simulink model "MultiUAV_DroneShow"  (R2026a)
settings: Solver=ode1  StopTime=74.3333  FixedStep=Ts_sim  MaxStep=0.01  AbsTol=1e-6
PreLoadFcn:
  | setupParams
values from neighbouring files (symbols this model uses):
  arm_duration = 2    [setupParams.m]
  gnss_deny_mask = false(N_uav, 1)    [setupParams.m]
  gnss_err_gain = sqrt(1 - gnss_err_pole^2)    [setupParams.m]
  gnss_err_pole = exp(-Ts_sim / gnss_err_tau)    [setupParams.m]
  gnss_err_seed = reshape(40000 + (1:(N_uav * 3)), N_uav, 3)    [setupParams.m]
  gps_accuracy_rtk_fix = 0.02    [setupParams.m]
  gps_lock_duration = 2    [setupParams.m]
  gravity = 9.81    [setupParams.m]
  hb_period_ticks = mavlink_hb_interval / Ts_sim    (= 100)    [setupParams.m]
  init_positions = init_positions(pad_of, :)    [planShow.m]    (also in setupParams.m = plan.init_positions)
  Kd_pos = repmat([Kd_xy Kd_xy Kd_z], N_uav, 1)    [setupParams.m]
  Kff_pos = Kd_pos    [setupParams.m]
  Kp_pos = repmat([Kp_xy Kp_xy Kp_z], N_uav, 1)    [setupParams.m]
  land_end_time = plan.land_end_time    [packShowUpload.m]    (also in planShow.m = show_flight_duration + land_duration; setupParams.m)
  land_speed = cfg.land_speed    [planShow.m]
  land_start_time = show_flight_duration    [planShow.m]    (also in setupParams.m = plan.land_start_time)
  land_total_duration = land_duration + land_settle    [planShow.m]    (also in setupParams.m = plan.land_total_duration)
  mav_sys_span = 250    [setupParams.m]
  N_uav = 20    [DroneShowExample.m]    (also in packShowUpload.m = cfg.N_uav; planShow.m = cfg.N_uav; setupParams.m = 10)
  num_waypoints = length(upload_times)    [packShowUpload.m]    (also in setupParams.m = pack.num_waypoints)
  rtcm_data_bytes = 180    [setupParams.m]
  rtcm_interval = 1.0    (= 1)    [setupParams.m]
  rtcm_payload_bytes = 4 * 4 * rtk_n_sat    [setupParams.m]
  rtcm_period_ticks = rtcm_interval / Ts_sim    (= 100)    [setupParams.m]
  rtk_amb_l1_base = 1000000 + mod(97 * (1:rtk_n_sat)', 1009)    [setupParams.m]
  rtk_amb_l1_rover = rtk_amb_l1_base + rtk_amb_l1    [setupParams.m]
  rtk_amb_l2_base = 1000000 + mod(89 * (1:rtk_n_sat)', 1009)    [setupParams.m]
  rtk_amb_l2_rover = rtk_amb_l2_base + rtk_amb_l2    [setupParams.m]
  rtk_base_lla = [42.3601, -71.0589, 10]    [setupParams.m]
  rtk_deny_mask = false(N_uav, 1)    [setupParams.m]
  rtk_f1 = 1575.42e6    (= 1575420000)    [setupParams.m]
  rtk_f2 = 1227.60e6    (= 1227600000)    [setupParams.m]
  rtk_fall_slew = -gps_accuracy_standard / reconverge_time    (= -0.3)    [setupParams.m]
  rtk_fix_thresh_l1 = 0.30    (= 0.3)    [setupParams.m]
  rtk_fix_thresh_wl = 0.25    [setupParams.m]
  rtk_inject_enable = double(~skip_preflight | rtk_deny_mask(:)')    [setupParams.m]
  rtk_lambda1 = rtk_c / rtk_f1    (= 0.190293672798)    [setupParams.m]
  rtk_lambda2 = rtk_c / rtk_f2    (= 0.244210213425)    [setupParams.m]
  rtk_lambda_wl = rtk_c / (rtk_f1 - rtk_f2)    (= 0.861918400322)    [setupParams.m]
  rtk_lock_dwell = 2.0    (= 2)    [setupParams.m]
  rtk_los = [cosd(rtk_el) .* sind(rtk_az), cosd(rtk_el) .* cosd(rtk_az), sind(rtk_el)]    [setupParams.m]
  rtk_mean_clk = zeros(2, 1)    [setupParams.m]
  rtk_mean_obs = zeros(2, rtk_n_sat)    [setupParams.m]
  rtk_n_sat = numel(rtk_az)    [setupParams.m]
  rtk_rough_range = pseudoranges(rtk_base_lla, rtk_sat_pos, 'RangeAccuracy', 0)    [setupParams.m]
  rtk_sat_pos = rtk_sat_pos_all(rtk_vis, :)    [setupParams.m]
  rtk_seedm_clk = 9101 + 8 * rtk_n_sat + (0:1)'    [setupParams.m]
  rtk_seedm_l1 = rtk_seedm_p2 + 2 * rtk_n_sat    [setupParams.m]
  rtk_seedm_l2 = rtk_seedm_l1 + 2 * rtk_n_sat    [setupParams.m]
  rtk_seedm_p1 = 9101 + reshape(0:2 * rtk_n_sat - 1, 2, rtk_n_sat)    [setupParams.m]
  rtk_seedm_p2 = rtk_seedm_p1 + 2 * rtk_n_sat    [setupParams.m]
  rtk_sigma_bp = [0, rtk_timeout, rtk_float_timeout]    [setupParams.m]
  rtk_sigma_table = sqrt(max(0, rtk_sigma_tiers.^2 - gps_accuracy_rtk_fix^2))    [setupParams.m]
  rtk_sigma_unfixed = 0.75    [setupParams.m]
  rtk_slip_thresh_l1 = 0.02    [setupParams.m]
  rtk_slip_thresh_wl = 0.10    (= 0.1)    [setupParams.m]
  rtk_status_l1 = 1    [setupParams.m]
  rtk_status_unfixed = 3    [setupParams.m]
  rtk_timeout = 2.5    [setupParams.m]
  rtk_var_clk = rtk_clock_sigma^2 * ones(2, 1)    [setupParams.m]
  rtk_var_l = [rtk_sigma_phase_base^2; rtk_sigma_phase_rover^2] * ones(1, rtk_n_sat)    [setupParams.m]
  rtk_var_p = [rtk_sigma_code_base^2;  rtk_sigma_code_rover^2 ] * ones(1, rtk_n_sat)    [setupParams.m]
  skip_preflight = traj_source == 1    [DroneShowExample.m]    (also in setupParams.m = false)
  st_period_ticks = mavlink_st_interval / Ts_sim    (= 100)    [setupParams.m]
  st_phase_ticks = st_period_ticks / 2    (= 50)    [setupParams.m]
  telemetry_tx_enable = double(~skip_preflight)    [setupParams.m]
  traj_upload_flat = zeros(N_uav*num_waypoints, 7)    [packShowUpload.m]    (also in setupParams.m = pack.traj_upload_flat)
  Ts_sim = cfg.Ts_sim    [packShowUpload.m]    (also in setupParams.m = 0.01)
  uav_loss_seed = 31000 + (1:N_uav)    [setupParams.m]
  uav_mass = 0.1    [setupParams.m]
  upload_duration = (total_packets + N_uav) * Ts_sim * 1.2    [packShowUpload.m]    (also in setupParams.m = pack.upload_duration)
  upload_rate_vec = [1 ./ upload_dt; 1 / upload_dt(end)]    [packShowUpload.m]    (also in setupParams.m = pack.upload_rate_vec)
  upload_request = traj_source == 2    [DroneShowExample.m]
undefined symbols (not defined in the file or in its folder): abort_request, DiscIntNeverNeededParam, doppler, loss_seed, packet_loss_rate, Payload, SystemID, uav_loss_rate
libraries: uavmavlinklib x22, hdlsllib x16, dspsigops x8, simulink x7, matrix_library x4, commchan3 x2, etargetslib x1, uavalgslib x1, sensorinslib x1, slpidlib x1, dspmathops x1, commrandsrc3 x1
(part 2 of 4)

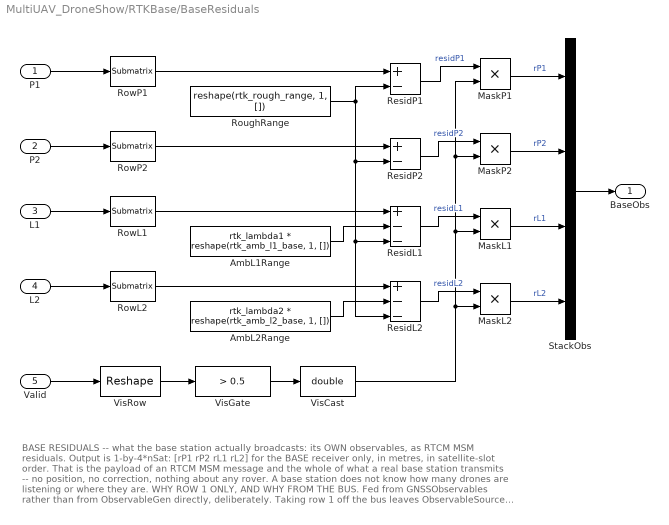
== system MultiUAV_DroneShow/RTKBase/BaseResiduals ==
  note: BASE RESIDUALS  --  what the base station actually broadcasts: its OWN observables, as RTCM MSM residuals.
      |
      | Output is 1-by-4*nSat: [rP1 rP2 rL1 rL2] for the BASE receiver only, in metres, in satellite-slot order.
      | That is the payload of an RTCM MSM message and the whole of what a real base station transmits -- no
      | position, no correction, nothing about any rover. A base station does not know how many drones are
      | listening or where they are.
      |
      | WHY ROW 1 ONLY, AND WHY FROM THE BUS. Fed from GNSSObservables rather than from ObservableGen directly,
      | deliberately. Taking row 1 off the bus leaves ObservableSource at one port, so both variant choices stay
      | identical and a RECORDING broadcasts its own base row exactly as the generator does -- the wire inherits
      | the source-agnosticism the engine itself was measured to have. Tapping ObservableGen would have added a
      | port to the Simulated choice only, and a divergence between the two choices is exactly the failure this
      | routing is arranged to make impossible.
      |
      | WHY RESIDUALS AND NOT THE OBSERVABLES. Raw values cannot survive the wire: at 2.47e7 m a single resolves
      | 2.000 m, and the payload is singles because 4*4*nSat = 128 bytes is what fits GPS_RTCM_DATA. So
      | each observable is differenced against rtk_rough_range, the clock-free noise-free base-to-satellite
      | range. A real rover can RECONSTRUCT that from the station position (RTCM 1005/1006) and the ephemeris,
      | which is what makes this a residual rather than data loss.
      |
      | WHY THE PHASE ROWS ARE ALSO CODE-ALIGNED. Subtracting the rough range alone is not enough: the base's
      | accumulated phase counter is ~1e6 cycles, so the phase residual would still sit at ~2.47e5 m, where a
      | single resolves 7.8e-3 m -- three and a half times COARSER than the 2.236e-3 m phase noise that has to
      | survive the trip. Folding the counter out here leaves ~2.3e3 m and 1.2e-4 m of resolution, nineteen times
      | finer than the noise and finer than MSM4's own 22-bit fine-phaserange field at 0.0005 m. Not a shortcut:
      | an MSM phaserange really is code-aligned, within metres of the pseudorange. The ~1e6-cycle counters are
      | RINEX semantics; this wire is RTCM semantics. Both directions were measured: residuals packed here,
      | and unpacked again the way a rover would.
      |
      | A rover differencing this recovers its OWN ambiguity rather than the between-receiver one, because the
      | base's contribution is already gone. That changes which integer a drone-side solve resolves, not whether
      | it can resolve one.
      |
      | INVISIBLE SLOTS CARRY ZERO -- that is what VisGate and the four Products are for. The payload is
      | fixed-width (nSat slots, always) because GPS_RTCM_DATA has no satellite-mask field to omit them with. An
      | unobserved slot's observable is 0 by the Valid contract, so differencing it would put -2.0e7 m on the
      | wire, indistinguishable from a catastrophically wrong residual. Masking to 0 keeps absent slots obviously
      | absent. The cost is that a slot whose residual is genuinely 0 looks absent -- a real limitation of a
      | mask-free payload, not a rounding concern: a residual is a clock plus noise, so exact 0 has measure zero.
      |
      | This was a MATLAB Function until 6-Sep-2026, and is now blocks. The replacement was accepted on two
      | measurements rather than on inspection: the block form produces bit-for-bit the same residuals the
      | function did, and at the same [1 0] rate; and the RTCM byte layout survives a round trip through these
      | very blocks. That round trip copies THIS subsystem into a throwaway model rather than restating the
      | formula anywhere it could silently drift out of step with what is built here.
  P1 : Inport
  P2 : Inport  Port=2
  L1 : Inport  Port=3
  L2 : Inport  Port=4
  Valid : Inport  Port=5
  AmbL1Range : Constant  Value=rtk_lambda1 * reshape(rtk_amb_l1_base, 1, [])  VectorParams1D=off
  AmbL2Range : Constant  Value=rtk_lambda2 * reshape(rtk_amb_l2_base, 1, [])  VectorParams1D=off
  MaskL1 : Product
  MaskL2 : Product
  MaskP1 : Product
  MaskP2 : Product
  ResidL1 : Sum  Inputs=+--
  ResidL2 : Sum  Inputs=+--
  ResidP1 : Sum  Inputs=+-
  ResidP2 : Sum  Inputs=+-
  RoughRange : Constant  Value=reshape(rtk_rough_range, 1, [])  VectorParams1D=off
  RowL1 : matrix_library/Submatrix  RowSpan=Range of rows  RowStartMode=Index  RowStartIndex=1  RowEndMode=Index  RowEndIndex=1  ColSpan=All columns  ColStartMode=First  ColStartIndex=1  ColEndMode=Last  ColEndIndex=1
  RowL2 : matrix_library/Submatrix  RowSpan=Range of rows  RowStartMode=Index  RowStartIndex=1  RowEndMode=Index  RowEndIndex=1  ColSpan=All columns  ColStartMode=First  ColStartIndex=1  ColEndMode=Last  ColEndIndex=1
  RowP1 : matrix_library/Submatrix  RowSpan=Range of rows  RowStartMode=Index  RowStartIndex=1  RowEndMode=Index  RowEndIndex=1  ColSpan=All columns  ColStartMode=First  ColStartIndex=1  ColEndMode=Last  ColEndIndex=1
  RowP2 : matrix_library/Submatrix  RowSpan=Range of rows  RowStartMode=Index  RowStartIndex=1  RowEndMode=Index  RowEndIndex=1  ColSpan=All columns  ColStartMode=First  ColStartIndex=1  ColEndMode=Last  ColEndIndex=1
  StackObs : Concatenate  NumInputs=4  Mode=Multidimensional array  ConcatenateDimension=2
  VisCast : DataTypeConversion  OutDataTypeStr=double  SaturateOnIntegerOverflow=off  RndMeth=Floor
  VisGate : simulink/Logic and Bit Operations/Compare To Constant  relop=>  const=0.5  OutDataTypeStr=boolean  ZeroCross=off
  VisRow : Reshape  OutputDimensionality=Row vector (2-D)
  BaseObs : Outport
  wires:
  P1/1 -> RowP1/1
  P2/1 -> RowP2/1
  L1/1 -> RowL1/1
  L2/1 -> RowL2/1
  Valid/1 -> VisRow/1
  VisRow/1 -> VisGate/1
  VisGate/1 -> VisCast/1
  RowP1/1 -> ResidP1/1
  RoughRange/1 -> ResidL1/3, ResidL2/3, ResidP2/2, ResidP1/2
  RowP2/1 -> ResidP2/1
  RowL1/1 -> ResidL1/1
  AmbL1Range/1 -> ResidL1/2
  RowL2/1 -> ResidL2/1
  AmbL2Range/1 -> ResidL2/2
  ResidP1/1 -> MaskP1/1  "residP1"
  VisCast/1 -> MaskP1/2, MaskP2/2, MaskL1/2, MaskL2/2
  ResidP2/1 -> MaskP2/1  "residP2"
  ResidL1/1 -> MaskL1/1  "residL1"
  ResidL2/1 -> MaskL2/1  "residL2"
  MaskP1/1 -> StackObs/1  "rP1"
  MaskP2/1 -> StackObs/2  "rP2"
  MaskL1/1 -> StackObs/3  "rL1"
  MaskL2/1 -> StackObs/4  "rL2"
  StackObs/1 -> BaseObs/1

== system MultiUAV_DroneShow/RTKBase/ObservableSource ==
  note: 1) Add Subsystem or Model blocks as valid variant choices.
      | 2) You cannot connect blocks at this level. At simulation, connectivity is automatically
      | determined, based on the active variant and port name matching.
  RoverPos : Inport
  Measured : Subsystem  Description=Recorded observables from rtk_measured_obs, e.g. a RINEX pair via rinexToObservables. The rover position input is unused here -- with real measurements the rover's truth is not known, and the observables already carry it.  VariantControl=rtk_obs_source == 2
  Simulated : Subsystem  Description=Today's simulated base station: pseudoranges() geometry, per-receiver clocks and noise, and the constellation from rtk_sat_pos.  VariantControl=rtk_obs_source == 1
  Obs : Outport

== system MultiUAV_DroneShow/RTKBase/RTKEngine ==
  Obs : Inport  Description=One epoch of raw GNSS observables, base row then rover row, metres. See createFleetBusObjects for the full contract.  OutDataTypeStr=Bus: GNSSObservableBus
  Cascade : MATLAB Function  TreatAsAtomicUnit=on
  SplitObs : BusSelector  OutputSignals=P1,P2,L1,L2,LOS,Valid
  Baseline : Outport
  Sigma : Outport  Port=2
  Status : Outport  Port=3
  Diag : Outport  Port=4
  wires:
  Cascade/1(Baseline) -> Baseline/1
  Cascade/2(Sigma) -> Sigma/1
  Cascade/3(Status) -> Status/1
  Cascade/4(Diag) -> Diag/1
  Obs/1 -> SplitObs/1
  SplitObs/1 -> Cascade/1(P1)  "<P1>"
  SplitObs/2 -> Cascade/2(P2)  "<P2>"
  SplitObs/3 -> Cascade/3(L1)  "<L1>"
  SplitObs/4 -> Cascade/4(L2)  "<L2>"
  SplitObs/5 -> Cascade/5(LOS)  "<LOS>"
  SplitObs/6 -> Cascade/6(Valid)  "<Valid>"

== system MultiUAV_DroneShow/RadioChannel/CorrectionAgeMonitor ==
  CorrAge : Inport
  GnssAvail : Inport  Port=2
  EngineSigma : Inport  Port=3
  ClampNonNegative : Saturate  UpperLimit=inf  LowerLimit=0  SampleTime=Ts_sim
  EngineGate : Product  SampleTime=Ts_sim
  EngineShortfall : Sqrt  SampleTime=Ts_sim
  EngineSigmaSq : Math  Operator=square  SampleTime=Ts_sim
  GnssAvailDbl : DataTypeConversion  OutDataTypeStr=double
  InjectEnable : Constant  Value=rtk_inject_enable
  InjectGate : Product
  InsFloorSq : Constant  Value=gps_accuracy_rtk_fix^2
  LogPosSigma : ToWorkspace  VariableName=posSigma  SaveFormat=Timeseries  SampleTime=-1
  ShortfallSq : Sum  Inputs=+-  SampleTime=Ts_sim
  SigmaGate : Product
  SigmaLUT : Lookup_n-D  NumberOfTableDimensions=1  BreakpointsForDimension1=rtk_sigma_bp  Table=rtk_sigma_table  InterpMethod=Flat  ExtrapMethod=Clip
  SigmaRateLimit : RateLimiter  RisingSlewLimit=inf  FallingSlewLimit=rtk_fall_slew  SampleTimeMode=inherited
  WorseOf : MinMax  Function=max  Inputs=2  SampleTime=Ts_sim
  PosSigma : Outport
  wires:
  InjectGate/1 -> LogPosSigma/1, PosSigma/1
  InjectEnable/1 -> InjectGate/2
  WorseOf/1 -> InjectGate/1
  CorrAge/1 -> SigmaLUT/1
  GnssAvail/1 -> GnssAvailDbl/1
  SigmaLUT/1 -> SigmaGate/1
  SigmaGate/1 -> SigmaRateLimit/1
  GnssAvailDbl/1 -> SigmaGate/2, EngineGate/2
  SigmaRateLimit/1 -> WorseOf/1
  EngineSigma/1 -> EngineSigmaSq/1
  EngineSigmaSq/1 -> ShortfallSq/1
  InsFloorSq/1 -> ShortfallSq/2
  ShortfallSq/1 -> ClampNonNegative/1  "sigma_shortfall_sq"
  ClampNonNegative/1 -> EngineShortfall/1
  EngineShortfall/1 -> EngineGate/1
  EngineGate/1 -> WorseOf/2

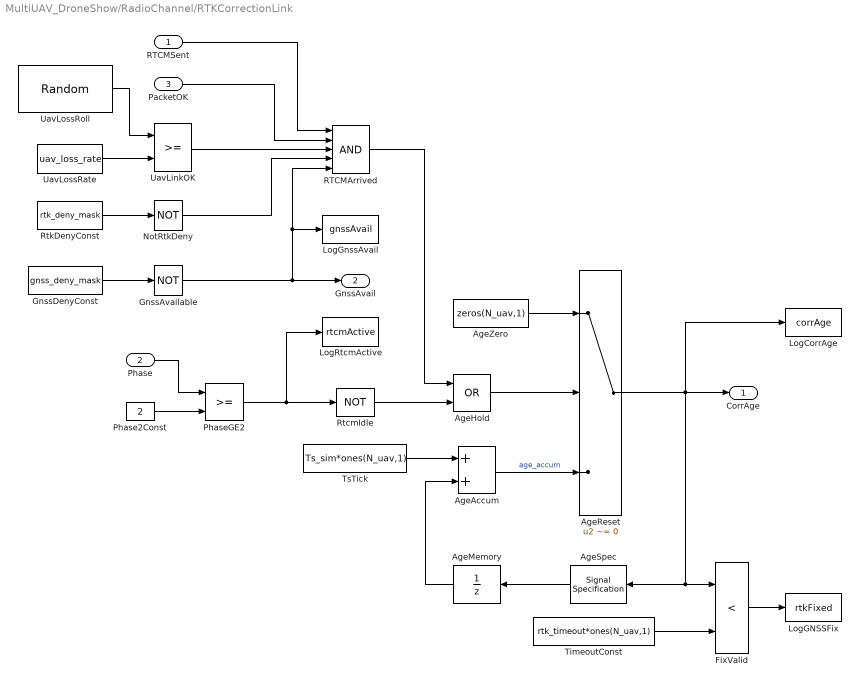
== system MultiUAV_DroneShow/RadioChannel/RTKCorrectionLink ==
  RTCMSent : Inport
  Phase : Inport  Port=2
  PacketOK : Inport  Port=3
  AgeAccum : Sum
  AgeHold : Logic  Operator=OR  AllPortsSameDT=off  OutDataTypeStr=boolean
  AgeMemory : UnitDelay  SampleTime=Ts_sim
  AgeReset : Switch  Criteria=u2 ~= 0  InputSameDT=off
  AgeSpec : SignalSpecification  OutDataTypeStr=double  Dimensions=N_uav  SampleTime=Ts_sim
  AgeZero : Constant  Value=zeros(N_uav,1)  OutDataTypeStr=double
  FixValid : RelationalOperator  Operator=<  OutDataTypeStr=boolean  InputSameDT=off
  GnssAvailable : Logic  Operator=NOT  Inputs=1
  GnssDenyConst : Constant  Value=gnss_deny_mask  SampleTime=Ts_sim
  LogCorrAge : ToWorkspace  VariableName=corrAge  SaveFormat=Timeseries  SampleTime=-1
  LogGNSSFix : ToWorkspace  VariableName=rtkFixed  SaveFormat=Timeseries  SampleTime=-1
  LogGnssAvail : ToWorkspace  VariableName=gnssAvail  SaveFormat=Timeseries  SampleTime=-1
  LogRtcmActive : ToWorkspace  VariableName=rtcmActive  SaveFormat=Timeseries  SampleTime=-1
  NotRtkDeny : Logic  Operator=NOT  Inputs=1
  Phase2Const : Constant  Value=2  SampleTime=Ts_sim
  PhaseGE2 : RelationalOperator  OutDataTypeStr=boolean  RndMeth=Simplest  InputSameDT=off
  RTCMArrived : Logic  Inputs=5  AllPortsSameDT=off  OutDataTypeStr=boolean
  RtcmIdle : Logic  Operator=NOT  Inputs=1  AllPortsSameDT=off  OutDataTypeStr=boolean
  RtkDenyConst : Constant  Value=rtk_deny_mask  SampleTime=Ts_sim
  TimeoutConst : Constant  Value=rtk_timeout*ones(N_uav,1)  OutDataTypeStr=double
  TsTick : Constant  Value=Ts_sim*ones(N_uav,1)  OutDataTypeStr=double
  UavLinkOK : RelationalOperator
  UavLossRate : Constant  Value=uav_loss_rate  SampleTime=Ts_sim
  UavLossRoll : UniformRandomNumber  Minimum=0  Seed=uav_loss_seed  SampleTime=Ts_sim
  CorrAge : Outport
  GnssAvail : Outport  Port=2
  wires:
  UavLossRoll/1 -> UavLinkOK/1
  RtkDenyConst/1 -> NotRtkDeny/1
  UavLossRate/1 -> UavLinkOK/2
  Phase/1 -> PhaseGE2/1
  GnssDenyConst/1 -> GnssAvailable/1
  Phase2Const/1 -> PhaseGE2/2
  AgeAccum/1 -> AgeReset/3  "age_accum"
  RTCMSent/1 -> RTCMArrived/1
  PhaseGE2/1 -> LogRtcmActive/1, RtcmIdle/1
  PacketOK/1 -> RTCMArrived/2
  UavLinkOK/1 -> RTCMArrived/3
  NotRtkDeny/1 -> RTCMArrived/4
  GnssAvailable/1 -> RTCMArrived/5, LogGnssAvail/1, GnssAvail/1
  RTCMArrived/1 -> AgeHold/1
  RtcmIdle/1 -> AgeHold/2
  TsTick/1 -> AgeAccum/1
  AgeZero/1 -> AgeReset/1
  AgeHold/1 -> AgeReset/2
  AgeMemory/1 -> AgeAccum/2
  AgeReset/1 -> LogCorrAge/1, CorrAge/1, AgeSpec/1, FixValid/1
  TimeoutConst/1 -> FixValid/2
  AgeSpec/1 -> AgeMemory/1
  FixValid/1 -> LogGNSSFix/1

== system MultiUAV_DroneShow/BaseStation/MissionProtocol/AddrJoinAck ==
  target_system : Inport
  target_component : Inport  Port=2
  AddI : Sum  OutDataTypeStr=uint32
  C_one : Constant  Value=uint32(1)  OutDataTypeStr=uint32
  C_span : Constant  Value=uint32(mav_sys_span)  OutDataTypeStr=uint32
  C_zero : Constant  Value=uint32(0)  OutDataTypeStr=uint32
  DTC_c32 : DataTypeConversion  OutDataTypeStr=uint32
  DTC_s32 : DataTypeConversion  OutDataTypeStr=uint32
  MaxC : MinMax  Function=max  Inputs=2  OutDataTypeStr=uint32
  MulB : Product  Inputs=**  OutDataTypeStr=uint32
  SubC : Sum  Inputs=+-|  OutDataTypeStr=uint32
  SwIdx : Switch  Criteria=u2 > Threshold
  idx : Outport
  wires:
  target_system/1 -> DTC_s32/1, SwIdx/2
  target_component/1 -> DTC_c32/1
  AddI/1 -> SwIdx/1
  DTC_s32/1 -> AddI/2
  C_span/1 -> MulB/2
  C_zero/1 -> SwIdx/3
  C_one/1 -> SubC/2, MaxC/2
  DTC_c32/1 -> MaxC/1
  SubC/1 -> MulB/1
  MulB/1 -> AddI/1
  MaxC/1 -> SubC/1
  SwIdx/1 -> idx/1

== system MultiUAV_DroneShow/BaseStation/MissionProtocol/AddrJoinReq ==
  target_system : Inport
  target_component : Inport  Port=2
  AddI : Sum  OutDataTypeStr=uint32
  C_one : Constant  Value=uint32(1)  OutDataTypeStr=uint32
  C_span : Constant  Value=uint32(mav_sys_span)  OutDataTypeStr=uint32
  C_zero : Constant  Value=uint32(0)  OutDataTypeStr=uint32
  DTC_c32 : DataTypeConversion  OutDataTypeStr=uint32
  DTC_s32 : DataTypeConversion  OutDataTypeStr=uint32
  MaxC : MinMax  Function=max  Inputs=2  OutDataTypeStr=uint32
  MulB : Product  Inputs=**  OutDataTypeStr=uint32
  SubC : Sum  Inputs=+-  OutDataTypeStr=uint32
  SwIdx : Switch  Criteria=u2 > Threshold
  idx : Outport
  wires:
  SwIdx/1 -> idx/1
  C_zero/1 -> SwIdx/3
  AddI/1 -> SwIdx/1
  DTC_s32/1 -> AddI/2
  MulB/1 -> AddI/1
  C_span/1 -> MulB/2
  SubC/1 -> MulB/1
  MaxC/1 -> SubC/1
  C_one/1 -> SubC/2, MaxC/2
  DTC_c32/1 -> MaxC/1
  target_component/1 -> DTC_c32/1
  target_system/1 -> SwIdx/2, DTC_s32/1

== system MultiUAV_DroneShow/BaseStation/MissionProtocol/MAckGate ==
  byteStreamInput : Inport
  Enable : EnablePort
  Deser_MAck : uavmavlinklib/MAVLink Deserializer  dialectSource=Select from standard MAVLink dialects  dialect=common.xml  dialectCustom=common.xml  version=2  messageType=MISSION_ACK  inputDataLength=off  SystemIDFilter=off  systemID=1  ComponentIDFilter=off  componentID=1  queueMsg=off  queueMsgSize=50  dropNum=off
  status : Outport  OutputWhenDisabled=reset  InitialOutput=0
  MsgOutput : Outport  Port=2
  wires:
  byteStreamInput/1 -> Deser_MAck/1
  Deser_MAck/1 -> status/1  "status"
  Deser_MAck/2 -> MsgOutput/1

== system MultiUAV_DroneShow/BaseStation/MissionProtocol/MReqGate ==
  byteStreamInput : Inport
  Enable : EnablePort
  Deser_MReq : uavmavlinklib/MAVLink Deserializer  dialectSource=Select from standard MAVLink dialects  dialect=common.xml  dialectCustom=common.xml  version=2  messageType=MISSION_REQUEST_INT  inputDataLength=off  SystemIDFilter=off  systemID=1  ComponentIDFilter=off  componentID=1  queueMsg=off  queueMsgSize=50  dropNum=off
  statusOutput : Outport  OutputWhenDisabled=reset  InitialOutput=0
  MsgOutput : Outport  Port=2
  wires:
  byteStreamInput/1 -> Deser_MReq/1
  Deser_MReq/1 -> statusOutput/1
  Deser_MReq/2 -> MsgOutput/1

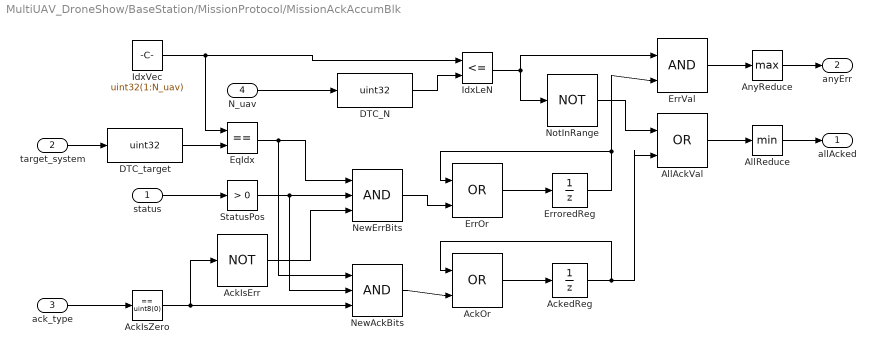
== system MultiUAV_DroneShow/BaseStation/MissionProtocol/MissionAckAccumBlk ==
  status : Inport
  target_system : Inport  Port=2
  ack_type : Inport  Port=3
  N_uav : Inport  Port=4
  AckIsErr : Logic  Operator=NOT  Inputs=1  IconShape=distinctive
  AckIsZero : hdlsllib/Logic and Bit Operations/Compare To Constant  relop===  const=uint8(0)  OutDataTypeStr=boolean
  AckOr : Logic  Operator=OR  IconShape=distinctive
  AckedReg : UnitDelay  InitialCondition=false(1,N_uav)  SampleTime=-1
  AllAckVal : Logic  Operator=OR  IconShape=distinctive
  AllReduce : MinMax
  AnyReduce : MinMax  Function=max
  DTC_N : DataTypeConversion  OutDataTypeStr=uint32
  DTC_target : DataTypeConversion  OutDataTypeStr=uint32
  EqIdx : RelationalOperator  Operator===
  ErrOr : Logic  Operator=OR  IconShape=distinctive
  ErrVal : Logic  IconShape=distinctive
  ErroredReg : UnitDelay  InitialCondition=false(1,N_uav)  SampleTime=-1
  IdxLeN : RelationalOperator  Operator=<=
  IdxVec : Constant  Value=uint32(1:N_uav)  OutDataTypeStr=uint32
  NewAckBits : Logic  Inputs=3  IconShape=distinctive
  NewErrBits : Logic  Inputs=3  IconShape=distinctive
  NotInRange : Logic  Operator=NOT  Inputs=1  IconShape=distinctive
  StatusPos : hdlsllib/Logic and Bit Operations/Compare To Constant  relop=>  const=0  OutDataTypeStr=boolean
  allAcked : Outport
  anyErr : Outport  Port=2
  wires:
  AnyReduce/1 -> anyErr/1
  AllReduce/1 -> allAcked/1
  ErrVal/1 -> AnyReduce/1
  AllAckVal/1 -> AllReduce/1
  NotInRange/1 -> AllAckVal/1
  IdxLeN/1 -> NotInRange/1, ErrVal/1
  DTC_N/1 -> IdxLeN/2
  ErrOr/1 -> ErroredReg/1
  NewErrBits/1 -> ErrOr/2
  ErroredReg/1 -> ErrOr/1, ErrVal/2
  AckOr/1 -> AckedReg/1
  NewAckBits/1 -> AckOr/2
  AckedReg/1 -> AckOr/1, AllAckVal/2
  AckIsErr/1 -> NewErrBits/3
  StatusPos/1 -> NewAckBits/2, NewErrBits/2
  EqIdx/1 -> NewAckBits/1, NewErrBits/1
  AckIsZero/1 -> AckIsErr/1, NewAckBits/3
  ack_type/1 -> AckIsZero/1
  status/1 -> StatusPos/1
  DTC_target/1 -> EqIdx/2
  IdxVec/1 -> EqIdx/1, IdxLeN/1
  N_uav/1 -> DTC_N/1
  target_system/1 -> DTC_target/1

== system MultiUAV_DroneShow/BaseStation/MissionProtocol/UploadIndexerBlk ==
  Phase : Inport
  UploadEnable : Inport  Port=2
  N_uav : Inport  Port=3
  num_waypoints : Inport  Port=4
  req_valid : Inport  Port=5
  req_ts : Inport  Port=6
  req_seq : Inport  Port=7
  UploadIndexerChart : Stateflow chart  TreatAsAtomicUnit=on
  mode : Outport
  mc_target : Outport  Port=2
  item_target : Outport  Port=3
  item_seq : Outport  Port=4
  lin_idx : Outport  Port=5
  give_up : Outport  Port=6
  wires:
  num_waypoints/1 -> UploadIndexerChart/4(num_waypoints)
  Phase/1 -> UploadIndexerChart/1(Phase)
  UploadIndexerChart/2(mc_target) -> mc_target/1
  req_seq/1 -> UploadIndexerChart/7(req_seq)
  UploadEnable/1 -> UploadIndexerChart/2(UploadEnable)
  req_ts/1 -> UploadIndexerChart/6(req_ts)
  req_valid/1 -> UploadIndexerChart/5(req_valid)
  N_uav/1 -> UploadIndexerChart/3(N_uav)
  UploadIndexerChart/1(mode) -> mode/1
  UploadIndexerChart/3(item_target) -> item_target/1
  UploadIndexerChart/4(item_seq) -> item_seq/1
  UploadIndexerChart/5(lin_idx) -> lin_idx/1
  UploadIndexerChart/6(give_up) -> give_up/1

== system MultiUAV_DroneShow/BaseStation/Transmitter/CommandLongTx ==
  In1 : Inport
  In2 : Inport  Port=2
  Enable : EnablePort
  BlankMsg_CL : uavmavlinklib/MAVLink Blank Message  dialectSource=Select from standard MAVLink dialects  dialect=common.xml  dialectCustom=common.xml  version=2  messageType=COMMAND_LONG  SystemID=1  ComponentID=1  SampleTime=inf
  Fill_CL : BusAssignment  AssignedSignals=Payload.command,Payload.target_system
  Pad_CL : dspsigops/Pad  padAlong=Rows  dimsToPad=1  valSrc=Specify via dialog  padVal=0  spec=Output size  padNumOutRowsSpecMethod=User-specified  numOutRows=1  padNumOutColsSpecMethod=User-specified  numOutCols=280  isVarDimsMode=off  padBeginning=0  padEnd=0  outSizeMode=User-specified  outSize=1  padSigAt=End  trunc_flag=None  roundingMode=Floor  overflowMode=off  truncOrWrapMode=Truncate  wrap_flag=None
  Ser_CL : uavmavlinklib/MAVLink Serializer  dialectSource=Select from standard MAVLink dialects  dialect=common.xml  dialectCustom=common.xml  version=2  messageType=COMMAND_LONG
  TermCL_len : Terminator
  Out1 : Outport
  wires:
  Pad_CL/1 -> Out1/1
  Fill_CL/1 -> Ser_CL/1
  BlankMsg_CL/1 -> Fill_CL/1
  Ser_CL/2 -> TermCL_len/1
  Ser_CL/1 -> Pad_CL/1
  In2/1 -> Fill_CL/3
  In1/1 -> Fill_CL/2

== system MultiUAV_DroneShow/BaseStation/Transmitter/HeartbeatTx ==
  Enable : EnablePort
  BlankMsg_HB : uavmavlinklib/MAVLink Blank Message  dialectSource=Select from standard MAVLink dialects  dialect=common.xml  dialectCustom=common.xml  version=2  messageType=HEARTBEAT  SystemID=1  ComponentID=1  SampleTime=inf
  Pad_HB : dspsigops/Pad  padAlong=Rows  dimsToPad=1  valSrc=Specify via dialog  padVal=0  spec=Output size  padNumOutRowsSpecMethod=User-specified  numOutRows=1  padNumOutColsSpecMethod=User-specified  numOutCols=280  isVarDimsMode=off  padBeginning=0  padEnd=0  outSizeMode=User-specified  outSize=1  padSigAt=End  trunc_flag=None  roundingMode=Floor  overflowMode=off  truncOrWrapMode=Truncate  wrap_flag=None
  Ser_HB : uavmavlinklib/MAVLink Serializer  dialectSource=Select from standard MAVLink dialects  dialect=common.xml  dialectCustom=common.xml  version=2  messageType=HEARTBEAT
  TermHB_len : Terminator
  Out1 : Outport
  wires:
  Pad_HB/1 -> Out1/1
  BlankMsg_HB/1 -> Ser_HB/1
  Ser_HB/2 -> TermHB_len/1
  Ser_HB/1 -> Pad_HB/1

== system MultiUAV_DroneShow/BaseStation/Transmitter/MissionCountTx ==
  In1 : Inport
  In2 : Inport  Port=2
  Enable : EnablePort
  AddrSplit : Subsystem
  BlankMsg_MC : uavmavlinklib/MAVLink Blank Message  dialectSource=Select from standard MAVLink dialects  dialect=common.xml  dialectCustom=common.xml  version=2  messageType=MISSION_COUNT  SystemID=1  ComponentID=1  SampleTime=inf
  Fill_MC : BusAssignment  AssignedSignals=Payload.count,Payload.target_system,Payload.target_component
  Pad_MC : dspsigops/Pad  padAlong=Rows  dimsToPad=1  valSrc=Specify via dialog  padVal=0  spec=Output size  padNumOutRowsSpecMethod=User-specified  numOutRows=1  padNumOutColsSpecMethod=User-specified  numOutCols=280  isVarDimsMode=off  padBeginning=0  padEnd=0  outSizeMode=User-specified  outSize=1  padSigAt=End  trunc_flag=None  roundingMode=Floor  overflowMode=off  truncOrWrapMode=Truncate  wrap_flag=None
  Ser_MC : uavmavlinklib/MAVLink Serializer  dialectSource=Select from standard MAVLink dialects  dialect=common.xml  dialectCustom=common.xml  version=2  messageType=MISSION_COUNT
  TermMC_len : Terminator
  Out1 : Outport
  wires:
  Pad_MC/1 -> Out1/1
  Fill_MC/1 -> Ser_MC/1
  BlankMsg_MC/1 -> Fill_MC/1
  Ser_MC/2 -> TermMC_len/1
  Ser_MC/1 -> Pad_MC/1
  In1/1 -> Fill_MC/2
  In2/1 -> AddrSplit/1(idx)
  AddrSplit/1(target_system) -> Fill_MC/3
  AddrSplit/2(target_component) -> Fill_MC/4

== system MultiUAV_DroneShow/BaseStation/Transmitter/MissionItemTx ==
  In1 : Inport
  In2 : Inport  Port=2
  In3 : Inport  Port=3
  In4 : Inport  Port=4
  In5 : Inport  Port=5
  Enable : EnablePort
  AddrSplit : Subsystem
  BlankMsg_MII : uavmavlinklib/MAVLink Blank Message  dialectSource=Select from standard MAVLink dialects  dialect=common.xml  dialectCustom=common.xml  version=2  messageType=MISSION_ITEM_INT  SystemID=1  ComponentID=1  SampleTime=inf
  C_mii_cmd : Constant  Value=16  OutDataTypeStr=uint16
  C_mii_frame : Constant  OutDataTypeStr=uint8
  Fill_MII : BusAssignment  AssignedSignals=Payload.target_system,Payload.seq,Payload.frame,Payload.command,Payload.x,Payload.y,Payload.z,Payload.target_component
  Pad_MII : dspsigops/Pad  padAlong=Rows  dimsToPad=1  valSrc=Specify via dialog  padVal=0  spec=Output size  padNumOutRowsSpecMethod=User-specified  numOutRows=1  padNumOutColsSpecMethod=User-specified  numOutCols=280  isVarDimsMode=off  padBeginning=0  padEnd=0  outSizeMode=User-specified  outSize=1  padSigAt=End  trunc_flag=None  roundingMode=Floor  overflowMode=off  truncOrWrapMode=Truncate  wrap_flag=None
  Ser_MII : uavmavlinklib/MAVLink Serializer  dialectSource=Select from standard MAVLink dialects  dialect=common.xml  dialectCustom=common.xml  version=2  messageType=MISSION_ITEM_INT
  TermMII_len : Terminator
  Out1 : Outport
  wires:
  C_mii_cmd/1 -> Fill_MII/5
  Ser_MII/1 -> Pad_MII/1
  C_mii_frame/1 -> Fill_MII/4
  BlankMsg_MII/1 -> Fill_MII/1
  In5/1 -> Fill_MII/8
  In4/1 -> Fill_MII/7
  In3/1 -> Fill_MII/6
  In2/1 -> Fill_MII/3
  Ser_MII/2 -> TermMII_len/1
  Fill_MII/1 -> Ser_MII/1
  Pad_MII/1 -> Out1/1
  In1/1 -> AddrSplit/1(idx)
  AddrSplit/1(target_system) -> Fill_MII/2
  AddrSplit/2(target_component) -> Fill_MII/9

== system MultiUAV_DroneShow/BaseStation/Transmitter/RTCMTx ==
  BaseObs : Inport
  In2 : Inport  Port=2
  Enable : EnablePort
  BlankMsg_RTCM : uavmavlinklib/MAVLink Blank Message  dialectSource=Select from standard MAVLink dialects  dialect=common.xml  dialectCustom=common.xml  version=2  messageType=GPS_RTCM_DATA  SystemID=1  ComponentID=1  SampleTime=inf
      link override ComponentIDConstant: Value=1
      link override MAVLinkMsgBusCreator: OutDataTypeStr=Bus: SL_Bus_MAVLink_GPS_RTCM_DATA_Packet
      link override MsgIDConstant: Value=233
      link override MsgModifier: SLBusName=SL_Bus_MAVLink_GPS_RTCM_DATA_Payload
      link override PayloadConstant: OutDataTypeStr=Bus: SL_Bus_MAVLink_GPS_RTCM_DATA_Payload
      link override SystemIDConstant: Value=1
  FillRTCM : BusAssignment  AssignedSignals=Payload.data,Payload.len
  PackRTKDataBlk : Subsystem
  Pad_RTCM : dspsigops/Pad  padAlong=Rows  dimsToPad=1  valSrc=Specify via dialog  padVal=0  spec=Output size  padNumOutRowsSpecMethod=User-specified  numOutRows=1  padNumOutColsSpecMethod=User-specified  numOutCols=194  isVarDimsMode=off  padBeginning=0  padEnd=0  outSizeMode=User-specified  outSize=1  padSigAt=End  trunc_flag=None  roundingMode=Floor  overflowMode=off  truncOrWrapMode=Truncate  wrap_flag=None
  Serializer_RTCM : uavmavlinklib/MAVLink Serializer  dialectSource=Select from standard MAVLink dialects  dialect=common.xml  dialectCustom=common.xml  version=2  messageType=GPS_RTCM_DATA
      link override MAVLinkEncoderBlock: SLBusName=SL_Bus_MAVLink_GPS_RTCM_DATA_Packet  MAVLinkMsg=GPS_RTCM_DATA  MsgMinLength=182  MsgMaxLength=182  MsgCRCValue=35
      link override SignalSpecification: OutDataTypeStr=Bus: SL_Bus_MAVLink_GPS_RTCM_DATA_Packet
  TermRTCMLen : Terminator
  Out1 : Outport
  wires:
  Serializer_RTCM/1 -> Pad_RTCM/1
  In2/1 -> FillRTCM/3
  BaseObs/1 -> PackRTKDataBlk/1(BaseObs)
  Pad_RTCM/1 -> Out1/1
  Serializer_RTCM/2 -> TermRTCMLen/1
  FillRTCM/1 -> Serializer_RTCM/1
  PackRTKDataBlk/1(data) -> FillRTCM/2
  BlankMsg_RTCM/1 -> FillRTCM/1

== system MultiUAV_DroneShow/BaseStation/Transmitter/SystemTimeTx ==
  In1 : Inport
  Enable : EnablePort
  BlankMsg_ST : uavmavlinklib/MAVLink Blank Message  dialectSource=Select from standard MAVLink dialects  dialect=common.xml  dialectCustom=common.xml  version=2  messageType=SYSTEM_TIME  SystemID=1  ComponentID=1  SampleTime=inf
  Fill_ST : BusAssignment  AssignedSignals=Payload.time_boot_ms
  Pad_ST : dspsigops/Pad  padAlong=Rows  dimsToPad=1  valSrc=Specify via dialog  padVal=0  spec=Output size  padNumOutRowsSpecMethod=User-specified  numOutRows=1  padNumOutColsSpecMethod=User-specified  numOutCols=280  isVarDimsMode=off  padBeginning=0  padEnd=0  outSizeMode=User-specified  outSize=1  padSigAt=End  trunc_flag=None  roundingMode=Floor  overflowMode=off  truncOrWrapMode=Truncate  wrap_flag=None
  Ser_ST : uavmavlinklib/MAVLink Serializer  dialectSource=Select from standard MAVLink dialects  dialect=common.xml  dialectCustom=common.xml  version=2  messageType=SYSTEM_TIME
  TermST_len : Terminator
  Out1 : Outport
  wires:
  Ser_ST/1 -> Pad_ST/1
  Fill_ST/1 -> Ser_ST/1
  BlankMsg_ST/1 -> Fill_ST/1
  Pad_ST/1 -> Out1/1
  Ser_ST/2 -> TermST_len/1
  In1/1 -> Fill_ST/2

== system MultiUAV_DroneShow/DroneFleet/Receiver/AddrJoin ==
  target_system : Inport
  target_component : Inport  Port=2
  AddI : Sum  OutDataTypeStr=uint32
  C_one : Constant  Value=uint32(1)  OutDataTypeStr=uint32
  C_span : Constant  Value=uint32(mav_sys_span)  OutDataTypeStr=uint32
  C_zero : Constant  Value=uint32(0)  OutDataTypeStr=uint32
  DTC_c32 : DataTypeConversion  OutDataTypeStr=uint32
  DTC_s32 : DataTypeConversion  OutDataTypeStr=uint32
  MaxC : MinMax  Function=max  Inputs=2  OutDataTypeStr=uint32
  MulB : Product  Inputs=**  OutDataTypeStr=uint32
  SubC : Sum  Inputs=+-  OutDataTypeStr=uint32
  SwIdx : Switch  Criteria=u2 > Threshold
  idx : Outport
  wires:
  target_system/1 -> DTC_s32/1, SwIdx/2
  target_component/1 -> DTC_c32/1
  DTC_c32/1 -> MaxC/1
  C_one/1 -> MaxC/2, SubC/2
  MaxC/1 -> SubC/1
  SubC/1 -> MulB/1
  C_span/1 -> MulB/2
  MulB/1 -> AddI/1
  DTC_s32/1 -> AddI/2
  AddI/1 -> SwIdx/1
  C_zero/1 -> SwIdx/3
  SwIdx/1 -> idx/1

== system MultiUAV_DroneShow/DroneFleet/Receiver/BufferWrite ==
  row_xyz : Inport
  lin_idx : Inport  Port=2
  Enable : EnablePort
  C_one_u8 : Constant  Value=uint8(1)  OutDataTypeStr=uint8
  WriteBuf : DataStoreWrite  DataStoreName=OnboardBuffer  EnableIndexing=on  NumberOfDimensions=2  IndexOptions=Index vector (port),Select all  Indices=,1  OutputSizes=1,3
  WriteFlag : DataStoreWrite  DataStoreName=ReceivedFlags  EnableIndexing=on  IndexOptions=Index vector (port)  Indices=1  OutputSizes=1
  wires:
  row_xyz/1 -> WriteBuf/1
  lin_idx/1 -> WriteFlag/2, WriteBuf/2
  C_one_u8/1 -> WriteFlag/1

== system MultiUAV_DroneShow/DroneFleet/Receiver/FlagsClearer ==
  Enable : EnablePort
  ClearWrite : DataStoreWrite  DataStoreName=ReceivedFlags  IndexOptions=Index vector (dialog)  Indices=1  OutputSizes=1
  ZerosVec : Constant  Value=zeros(N_uav*num_waypoints,1,'uint8')  OutDataTypeStr=uint8
  wires:
  ZerosVec/1 -> ClearWrite/1

== system MultiUAV_DroneShow/DroneFleet/Receiver/MIGate ==
  byteStreamInput : Inport
  Enable : EnablePort
  Deser_MI : uavmavlinklib/MAVLink Deserializer  dialectSource=Select from standard MAVLink dialects  dialect=common.xml  dialectCustom=common.xml  version=2  messageType=MISSION_ITEM_INT  inputDataLength=off  SystemIDFilter=off  systemID=1  ComponentIDFilter=off  componentID=1  queueMsg=off  queueMsgSize=50  dropNum=off
  status : Outport  OutputWhenDisabled=reset  InitialOutput=0
  MsgOutput : Outport  Port=2
  wires:
  byteStreamInput/1 -> Deser_MI/1
  Deser_MI/1 -> status/1  "status"
  Deser_MI/2 -> MsgOutput/1

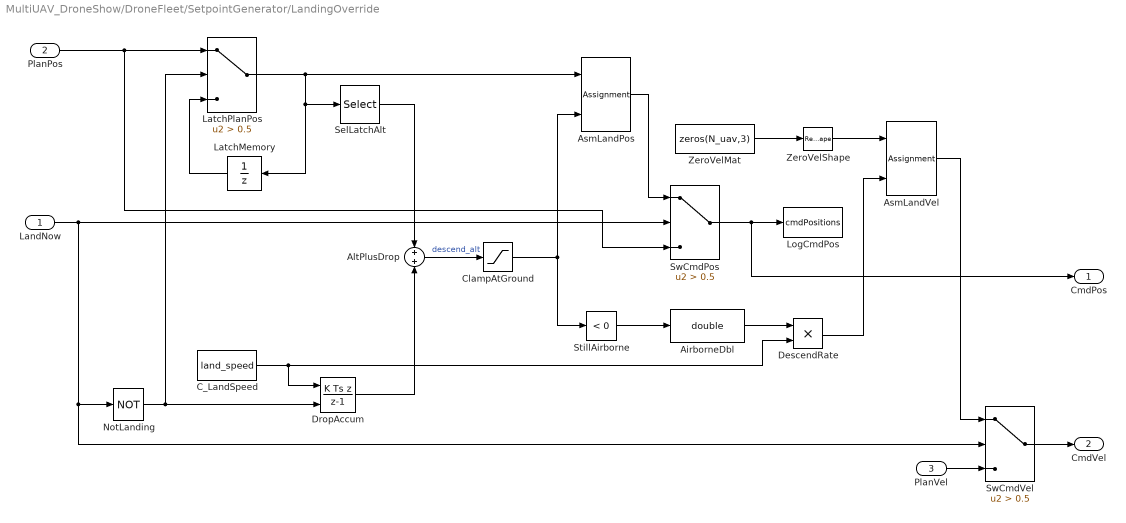
== system MultiUAV_DroneShow/DroneFleet/SetpointGenerator/LandingOverride ==
  LandNow : Inport
  PlanPos : Inport  Port=2
  PlanVel : Inport  Port=3
  AirborneDbl : DataTypeConversion  OutDataTypeStr=double  SaturateOnIntegerOverflow=off  RndMeth=Floor
  AltPlusDrop : Sum
  AsmLandPos : Assignment  NumberOfDimensions=2  IndexOptions=Assign all,Index vector (dialog)  Indices=,3  OutputSizes=1,1
  AsmLandVel : Assignment  NumberOfDimensions=2  IndexOptions=Assign all,Index vector (dialog)  Indices=,3  OutputSizes=1,1
  C_LandSpeed : Constant  Value=land_speed  SampleTime=Ts_sim
  ClampAtGround : Saturate  UpperLimit=0  LowerLimit=-inf
  DescendRate : Product
  DropAccum : DiscreteIntegrator  IntegratorMethod=Integration: Backward Euler  gainval=1  ExternalReset=level  SampleTime=Ts_sim  ICPrevOutput=DiscIntNeverNeededParam  ICPrevScaledInput=DiscIntNeverNeededParam
  LatchMemory : UnitDelay  SampleTime=Ts_sim
  LatchPlanPos : Switch  Criteria=u2 > Threshold  Threshold=0.5
  LogCmdPos : ToWorkspace  VariableName=cmdPositions  SaveFormat=Timeseries  SampleTime=-1
  NotLanding : Logic  Operator=NOT  AllPortsSameDT=off  OutDataTypeStr=boolean
  SelLatchAlt : Selector  NumberOfDimensions=2  IndexOptions=Select all,Index vector (dialog)  Indices=,3  OutputSizes=1,1
  StillAirborne : hdlsllib/Logic and Bit Operations/Compare To Zero  relop=<  OutDataTypeStr=boolean
  SwCmdPos : Switch  Criteria=u2 > Threshold  Threshold=0.5
  SwCmdVel : Switch  Criteria=u2 > Threshold  Threshold=0.5
  ZeroVelMat : Constant  Value=zeros(N_uav,3)
  ZeroVelShape : Reshape  OutputDimensionality=Customize  OutputDimensions=[N_uav 3]
  CmdPos : Outport
  CmdVel : Outport  Port=2
  wires:
  LandNow/1 -> SwCmdPos/2, NotLanding/1, SwCmdVel/2
  NotLanding/1 -> DropAccum/2, LatchPlanPos/2
  PlanPos/1 -> LatchPlanPos/1, SwCmdPos/3
  DropAccum/1 -> AltPlusDrop/2
  LatchPlanPos/1 -> SelLatchAlt/1, LatchMemory/1, AsmLandPos/1
  SwCmdVel/1 -> CmdVel/1
  SelLatchAlt/1 -> AltPlusDrop/1
  LatchMemory/1 -> LatchPlanPos/3
  C_LandSpeed/1 -> DropAccum/1, DescendRate/2
  AltPlusDrop/1 -> ClampAtGround/1  "descend_alt"
  ClampAtGround/1 -> AsmLandPos/2, StillAirborne/1
  AsmLandPos/1 -> SwCmdPos/1
  StillAirborne/1 -> AirborneDbl/1
  ZeroVelMat/1 -> ZeroVelShape/1
  SwCmdPos/1 -> LogCmdPos/1, CmdPos/1
  AirborneDbl/1 -> DescendRate/1
  ZeroVelShape/1 -> AsmLandVel/1
  DescendRate/1 -> AsmLandVel/2
  AsmLandVel/1 -> SwCmdVel/1
  PlanVel/1 -> SwCmdVel/3

== system MultiUAV_DroneShow/DroneFleet/SetpointGenerator/PlannedTrajectory ==
  ShowTime : Inport
  OnboardTrajSource : Subsystem
  SelPos : Selector  NumberOfDimensions=2  IndexOptions=Index vector (dialog),Select all  Indices=[1 2 3],1  OutputSizes=3,10
  SelVel : Selector  NumberOfDimensions=2  IndexOptions=Index vector (dialog),Select all  Indices=[4 5 6],1  OutputSizes=3,10
  SelYaw : Selector  NumberOfDimensions=2  IndexOptions=Index vector (dialog),Select all  Indices=7,1  OutputSizes=1,10
  TrajReshape : Reshape  OutputDimensionality=Customize  OutputDimensions=[7 N_uav]
  TrajSourceFleet : FromWorkspace  VariableName=traj_show_ts  SampleTime=Ts_sim  OutputAfterFinalValue=Holding final value
  TrajTransPos : Math  Operator=transpose
  TrajTransVel : Math  Operator=transpose
  TrajTransYaw : Math  Operator=transpose
  TrajVariant : VariantSource  ShowConditionOnBlock=on  VariantControls={traj_source == 1, traj_source == 2}
  ZOH_PlanPos : ZeroOrderHold  SampleTime=Ts_sim
  ZOH_PlanVel : ZeroOrderHold  SampleTime=Ts_sim
  PlanPos : Outport
  PlanVel : Outport  Port=2
  PlanYaw : Outport  Port=3
  wires:
  ShowTime/1 -> OnboardTrajSource/1(ShowTime)  "show_time"
  ZOH_PlanVel/1 -> PlanVel/1
  ZOH_PlanPos/1 -> PlanPos/1
  TrajTransVel/1 -> ZOH_PlanVel/1
  TrajTransPos/1 -> ZOH_PlanPos/1
  SelVel/1 -> TrajTransVel/1
  SelPos/1 -> TrajTransPos/1
  TrajVariant/1 -> SelVel/1, SelPos/1, SelYaw/1  "target_traj"
  OnboardTrajSource/1(TrajMatrix) -> TrajVariant/2
  SelYaw/1 -> TrajTransYaw/1
  TrajReshape/1 -> TrajVariant/1
  TrajSourceFleet/1 -> TrajReshape/1
  TrajTransYaw/1 -> PlanYaw/1

== system MultiUAV_DroneShow/DroneFleet/Transmitter/DownlinkMux ==
  ReqBytes : Inport
  ReqPending : Inport  Port=2
  AckBytes : Inport  Port=3
  AckActive : Inport  Port=4
  TelemetryBytes : Inport  Port=5
  Sw_MAckOut : Switch  Criteria=u2 > Threshold  Threshold=0.5
  Sw_MReqOut : Switch  Criteria=u2 > Threshold  Threshold=0.5  SaturateOnIntegerOverflow=off  InputSameDT=off
  MAVLinkBytes : Outport
  wires:
  TelemetryBytes/1 -> Sw_MReqOut/3
  ReqBytes/1 -> Sw_MReqOut/1
  AckActive/1 -> Sw_MAckOut/2
  ReqPending/1 -> Sw_MReqOut/2
  Sw_MAckOut/1 -> MAVLinkBytes/1
  AckBytes/1 -> Sw_MAckOut/1
  Sw_MReqOut/1 -> Sw_MAckOut/3

== system MultiUAV_DroneShow/DroneFleet/Transmitter/MissionAckEncoder ==
  AckTrigger : Inport
  AckActiveAnd : Logic
  AckCounter : DiscreteIntegrator  gainval=1/Ts_sim  SampleTime=Ts_sim  LimitOutput=on  UpperSaturationLimit=double(N_uav)+1  LowerSaturationLimit=0  ICPrevOutput=DiscIntNeverNeededParam  ICPrevScaledInput=DiscIntNeverNeededParam
  AckMsgGate : Subsystem
  ActiveToDbl : DataTypeConversion  OutDataTypeStr=double
  CntGe1 : RelationalOperator
  CntLeN : RelationalOperator  Operator=<=
  CntOne : Constant  OutDataTypeStr=double
  MinCntN : MinMax  Inputs=2
  MulTargetSys : Product
  NuavConst : Constant  Value=uint8(N_uav)  OutDataTypeStr=uint8
  NuavToDbl : DataTypeConversion  OutDataTypeStr=double
  TargetSysToU8 : DataTypeConversion  OutDataTypeStr=uint16
  AckBytes : Outport
  AckActive : Outport  Port=2
  wires:
  AckCounter/1 -> MinCntN/1, CntLeN/1, CntGe1/1
  CntOne/1 -> CntGe1/2
  AckTrigger/1 -> AckCounter/1
  NuavToDbl/1 -> MinCntN/2, CntLeN/2
  NuavConst/1 -> NuavToDbl/1
  MinCntN/1 -> MulTargetSys/1
  CntLeN/1 -> AckActiveAnd/2
  CntGe1/1 -> AckActiveAnd/1
  AckActiveAnd/1 -> ActiveToDbl/1, AckMsgGate/Enable, AckActive/1
  ActiveToDbl/1 -> MulTargetSys/2
  MulTargetSys/1 -> TargetSysToU8/1
  TargetSysToU8/1 -> AckMsgGate/1(In1)
  AckMsgGate/1(Out1) -> AckBytes/1

== system MultiUAV_DroneShow/DroneFleet/Transmitter/MissionRequestEncoder ==
  RxTargetSys : Inport
  MissionFlags : Inport  Port=2
  RxStatus : Inport  Port=3
  DTC_ReqTs_u8 : DataTypeConversion  OutDataTypeStr=uint16  SaturateOnIntegerOverflow=off  RndMeth=Floor
  ReqActive : Logic  AllPortsSameDT=off  OutDataTypeStr=boolean
  ReqCountLeading : Sum  Inputs=+
  ReqIsSet : hdlsllib/Logic and Bit Operations/Compare To Constant  relop=~=  const=0  OutDataTypeStr=boolean
  ReqLeadingRun : dspmathops/Cumulative Product  dim=Columns  InputProcessing=Columns as channels (frame based)  reset_popup=None  roundingMode=Floor  overflowMode=off  outputMin=[]  outputMax=[]
  ReqMsgGate : Subsystem
  ReqNwpConst : Constant  Value=num_waypoints  OutDataTypeStr=uint16
  ReqSelCol : Selector  NumberOfDimensions=2  IndexOptions=Select all,Index vector (port)  Indices=,  OutputSizes=1,1
  ReqSeqU16 : DataTypeConversion  OutDataTypeStr=uint16  SaturateOnIntegerOverflow=off  RndMeth=Floor
  ReqSetDbl : DataTypeConversion  OutDataTypeStr=double  SaturateOnIntegerOverflow=off  RndMeth=Floor
  ReqSwSeq : Switch  Criteria=u2 > Threshold  Threshold=0.5
  ReqTsClamp : Saturate  UpperLimit=N_uav  LowerLimit=1
  ReqTsValid : hdlsllib/Logic and Bit Operations/Interval Test  IntervalClosedRight=on  uplimit=N_uav  IntervalClosedLeft=on  lowlimit=1  OutDataTypeStr=boolean
  ReqBytes : Outport
  ReqPending : Outport  Port=2
  wires:
  ReqIsSet/1 -> ReqSetDbl/1
  RxTargetSys/1 -> DTC_ReqTs_u8/1, ReqTsClamp/1, ReqTsValid/1
  ReqSelCol/1 -> ReqIsSet/1
  MissionFlags/1 -> ReqSelCol/1
  ReqTsClamp/1 -> ReqSelCol/2
  RxStatus/1 -> ReqActive/1
  ReqTsValid/1 -> ReqSwSeq/2, ReqActive/2
  ReqActive/1 -> ReqPending/1, ReqMsgGate/Enable
  ReqSetDbl/1 -> ReqLeadingRun/1
  ReqLeadingRun/1 -> ReqCountLeading/1
  ReqCountLeading/1 -> ReqSeqU16/1  "req_count"
  ReqSeqU16/1 -> ReqSwSeq/1
  ReqNwpConst/1 -> ReqSwSeq/3
  DTC_ReqTs_u8/1 -> ReqMsgGate/1(In1)
  ReqSwSeq/1 -> ReqMsgGate/2(In2)
  ReqMsgGate/1(Out1) -> ReqBytes/1

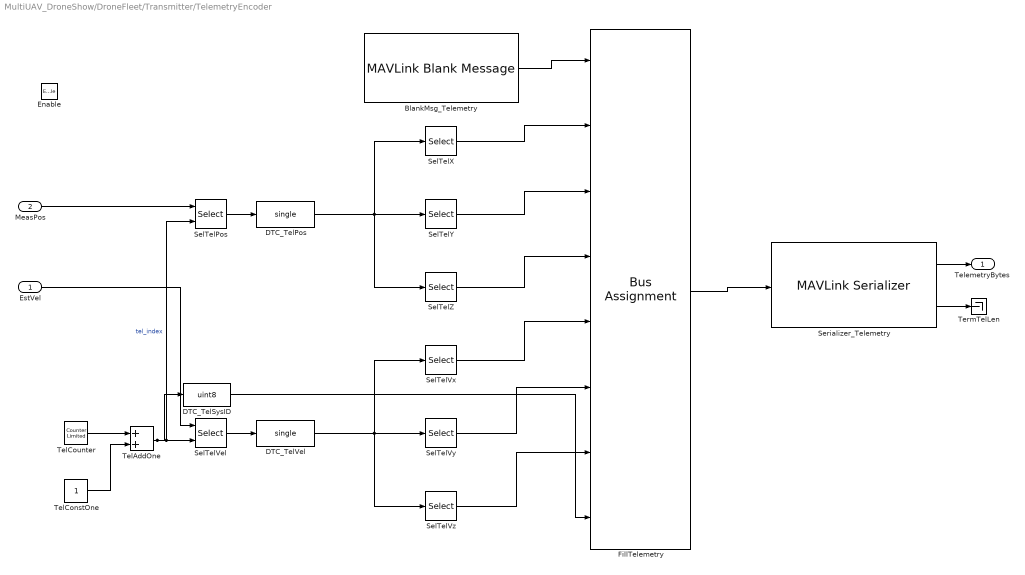
== system MultiUAV_DroneShow/DroneFleet/Transmitter/TelemetryEncoder ==
  EstVel : Inport
  MeasPos : Inport  Port=2
  Enable : EnablePort
  BlankMsg_Telemetry : uavmavlinklib/MAVLink Blank Message  dialectSource=Select from standard MAVLink dialects  dialect=common.xml  dialectCustom=common.xml  version=2  messageType=LOCAL_POSITION_NED  SystemID=1  ComponentID=1  SampleTime=inf
  DTC_TelPos : DataTypeConversion  OutDataTypeStr=single  SaturateOnIntegerOverflow=off  RndMeth=Floor
  DTC_TelSysID : DataTypeConversion  OutDataTypeStr=uint8  SaturateOnIntegerOverflow=off  RndMeth=Floor
  DTC_TelVel : DataTypeConversion  OutDataTypeStr=single  SaturateOnIntegerOverflow=off  RndMeth=Floor
  FillTelemetry : BusAssignment  AssignedSignals=Payload.x,Payload.y,Payload.z,Payload.vx,Payload.vy,Payload.vz,SystemID
  SelTelPos : Selector  NumberOfDimensions=2  InputPortWidth=3  IndexOptions=Index vector (port),Select all  Indices=1,1  OutputSizes=1
  SelTelVel : Selector  NumberOfDimensions=2  InputPortWidth=3  IndexOptions=Index vector (port),Select all  Indices=1,1  OutputSizes=1
  SelTelVx : Selector  InputPortWidth=3  IndexOptions=Index vector (dialog)  Indices=1  OutputSizes=1
  SelTelVy : Selector  InputPortWidth=3  IndexOptions=Index vector (dialog)  Indices=2  OutputSizes=1
  SelTelVz : Selector  InputPortWidth=3  IndexOptions=Index vector (dialog)  Indices=3  OutputSizes=1
  SelTelX : Selector  InputPortWidth=3  IndexOptions=Index vector (dialog)  Indices=1  OutputSizes=1
  SelTelY : Selector  InputPortWidth=3  IndexOptions=Index vector (dialog)  Indices=2  OutputSizes=1
  SelTelZ : Selector  InputPortWidth=3  IndexOptions=Index vector (dialog)  Indices=3  OutputSizes=1
  Serializer_Telemetry : uavmavlinklib/MAVLink Serializer  dialectSource=Select from standard MAVLink dialects  dialect=common.xml  dialectCustom=common.xml  version=2  messageType=LOCAL_POSITION_NED
  TelAddOne : Sum
  TelConstOne : Constant
  TelCounter : simulink/Sources/Counter Limited  uplimit=N_uav-1  tsamp=-1
  TermTelLen : Terminator
  TelemetryBytes : Outport
  wires:
  TelCounter/1 -> TelAddOne/1
  SelTelX/1 -> FillTelemetry/2
  TelConstOne/1 -> TelAddOne/2
  MeasPos/1 -> SelTelPos/1
  TelAddOne/1 -> SelTelVel/2, SelTelPos/2, DTC_TelSysID/1  "tel_index"
  EstVel/1 -> SelTelVel/1
  SelTelVel/1 -> DTC_TelVel/1
  SelTelPos/1 -> DTC_TelPos/1
  DTC_TelPos/1 -> SelTelX/1, SelTelY/1, SelTelZ/1
  DTC_TelVel/1 -> SelTelVx/1, SelTelVz/1, SelTelVy/1
  BlankMsg_Telemetry/1 -> FillTelemetry/1
  SelTelVz/1 -> FillTelemetry/7
  SelTelY/1 -> FillTelemetry/3
  SelTelZ/1 -> FillTelemetry/4
  SelTelVx/1 -> FillTelemetry/5
  SelTelVy/1 -> FillTelemetry/6
  FillTelemetry/1 -> Serializer_Telemetry/1
  Serializer_Telemetry/1 -> TelemetryBytes/1
  Serializer_Telemetry/2 -> TermTelLen/1
  DTC_TelSysID/1 -> FillTelemetry/8

== system MultiUAV_DroneShow/RTKBase/ObservableSource/Measured ==
  RoverPos : Inport
  FromRecording : FromWorkspace  VariableName=rtk_measured_obs  OutDataTypeStr=Bus: GNSSObservableBus  SampleTime=rtcm_interval  Interpolate=off  OutputAfterFinalValue=Holding final value
  UnusedRoverPos : Terminator
  Obs : Outport
  wires:
  RoverPos/1 -> UnusedRoverPos/1
  FromRecording/1 -> Obs/1

== system MultiUAV_DroneShow/RTKBase/ObservableSource/Simulated ==
  RoverPos : Inport
  BusObs : BusCreator  Inputs=6  OutDataTypeStr=Bus: GNSSObservableBus
  ObservableGen : Subsystem
  SatLOS : Constant  Value=rtk_los  SampleTime=rtcm_interval
  SatValid : Constant  Value=ones(rtk_n_sat, 1)  SampleTime=rtcm_interval
  Obs : Outport
  wires:
  RoverPos/1 -> ObservableGen/1(RoverPos)
  ObservableGen/1(P1) -> BusObs/1  "P1"
  ObservableGen/2(P2) -> BusObs/2  "P2"
  ObservableGen/3(L1) -> BusObs/3  "L1"
  ObservableGen/4(L2) -> BusObs/4  "L2"
  SatLOS/1 -> BusObs/5  "LOS"
  SatValid/1 -> BusObs/6  "Valid"
  BusObs/1 -> Obs/1

== system MultiUAV_DroneShow/BaseStation/Transmitter/MissionCountTx/AddrSplit ==
  idx : Inport
  AddC1 : Sum  OutDataTypeStr=uint16
  AddS1 : Sum  OutDataTypeStr=uint16
  C_one : Constant  Value=uint16(1)  OutDataTypeStr=uint16
  C_span : Constant  Value=uint16(mav_sys_span)  OutDataTypeStr=uint16
  C_zero : Constant  Value=uint8(0)  OutDataTypeStr=uint8
  DTC_comp : DataTypeConversion  OutDataTypeStr=uint8
  DTC_sys : DataTypeConversion  OutDataTypeStr=uint8
  DivF : Product  Inputs=*/  OutDataTypeStr=uint16
  MaxIdx : MinMax  Function=max  Inputs=2  OutDataTypeStr=uint16
  MulS : Product  Inputs=**  OutDataTypeStr=uint16
  Sub1 : Sum  Inputs=+-  OutDataTypeStr=uint16
  SubS : Sum  Inputs=+-  OutDataTypeStr=uint16
  SwComp : Switch  Criteria=u2 > Threshold
  SwSys : Switch  Criteria=u2 > Threshold
  target_system : Outport
  target_component : Outport  Port=2
  wires:
  SwComp/1 -> target_component/1
  SwSys/1 -> target_system/1
  DTC_comp/1 -> SwComp/1
  C_zero/1 -> SwComp/3, SwSys/3
  DTC_sys/1 -> SwSys/1
  AddC1/1 -> DTC_comp/1
  AddS1/1 -> DTC_sys/1
  SubS/1 -> AddS1/1
  MulS/1 -> SubS/2
  DivF/1 -> AddC1/1, MulS/1
  C_span/1 -> MulS/2, DivF/2
  Sub1/1 -> SubS/1, DivF/1
  MaxIdx/1 -> Sub1/1
  C_one/1 -> AddC1/2, AddS1/2, Sub1/2, MaxIdx/2
  idx/1 -> SwComp/2, SwSys/2, MaxIdx/1
